simulink library "adv_mosfet"  (R2025b)
settings: Solver=VariableStepAuto  StartTime=0.0  StopTime=10.0  RelTol=1e-3
undefined symbols (not defined in the file): mosfet, Rgate_turn_off, Rgate_turn_on
libraries: fl_lib x8, nesl_utility x6, advanced_mosfet_lib x1
settings Model: Creator=dbagn  LastModifiedBy=dbagn

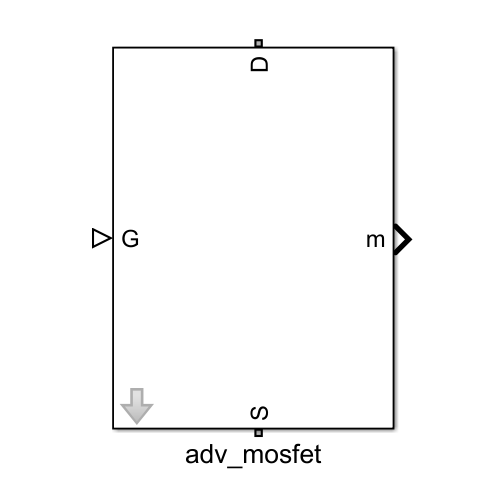
[thumbnail: Simulink's stored preview of the top-level diagram]
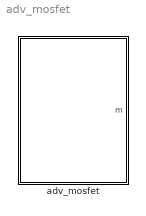
== system adv_mosfet ==
  adv_mosfet : Subsystem  mask{Rds_on_m=mosfet.inv.Rds_on, Vth_m=mosfet.inv.Vth, Vdon_diode_m=mosfet.inv.Vdon_diode, Rdon_diode_m=mosfet.inv.Rdon_diode, g_fs_m=mosfet.inv.g_fs, Cgs_m=mosfet.inv.Cgs, Cgd_m=mosfet.inv.Cgd, Cds_m=mosfet.inv.Cds, Eon_m=mosfet.inv.Eon, Eoff_m=mosfet.inv.Eoff, Err_m=mosfet.inv.Erec, Voff_sw_loss_m=mosfet.inv.Voff_sw_losses, Ion_sw_loss_m=mosfet.inv.Ion_sw_losses, Rgate_internal_m=mosfet.inv.Rgate_internal, Rgate_turn_on_m=Rgate_turn_on, Rgate_turn_off_m=Rgate_turn_off, Lstray_m=mosfet.inv.Lstray_module, Ld=mosfet.inv.Ld, RLd=mosfet.inv.RLd, Ls=mosfet.inv.Ls, RLs=mosfet.inv.RLs}
      mask prompts: Rds_on_m "Rds_on (Ohm)"; Vth_m "Vth (V)"; Vdon_diode_m "Vdon_diode (V)"; Rdon_diode_m "Rdon_diode (Ohm)"; g_fs_m "g_fs (A/V)"; Cgs_m "Cgs (F)"; Cgd_m "Cgd (F)"; Cds_m "Cds (F)"; Eon_m "Eon (J)"; Eoff_m "Eoff (J)"; Err_m "Err (J)"; Voff_sw_loss_m "Voff_sw_loss (V)"; Ion_sw_loss_m "Ion _sw_loss (A)"; Rgate_internal_m "Rgate internal (Ohm)"; Rgate_turn_on_m "Rgate turn on (Ohm)"; Rgate_turn_off_m "Rgate turn off (Ohm)"; Lstray_m "Lstray module (H)"; Ld "Ld (H)"; RLd "RLd (Ohm)"; Ls "Ls (H)"; RLs "RLs (Ohm)"
      settings: PortSchema="{\"entries\":[{\"content\":{\"sides\":[{\"content\":{\"connectorIds\":[\"LConn1\"]},\"type\":\"ConnectorPlacement.EquallySpacedRectSide\",\"uuid\":\"325dc963-858c-47f0-8995-f323ab4d9c46\"},{\"content\":{\"connectorIds\":[\"Out1\"],\"side\":\"RIGHT\"},\"type\":\"ConnectorPlacement.EquallySpacedRectSide\",\"uuid\":\"e9e66084-ecb2-40fb-9a1e-77677e0cc1df\"},{\"content\":{\"connectorIds\":[\"LConn2\"],\"side\":\"TOP\"},\"type\":\"ConnectorPlacement.EquallySpacedRectSide\",\"uuid\":\"9480d797-f2f6-459b-bb7c-d63861b57fde\"},{\"content\":{\"connectorIds\":[\"RConn1\"],\"side\":\"BOTTOM\"},\"type\":\"ConnectorPlacement.EquallySpacedRectSide\",\"uuid\":\"b13176d9-73b9-4822-9a0d-ec75065272bc\"}]},\"type\":\"ConnectorPlacement.EquallySpacedConnector\",\"uuid\":\"5e4a07d9-f5e8-4613-9049-5a866b5d2453\"}],\"packageUris\":[\"http://schema.mathworks.com/mf0/Connector/R2020b\"],\"version\":\"1.0\"}"

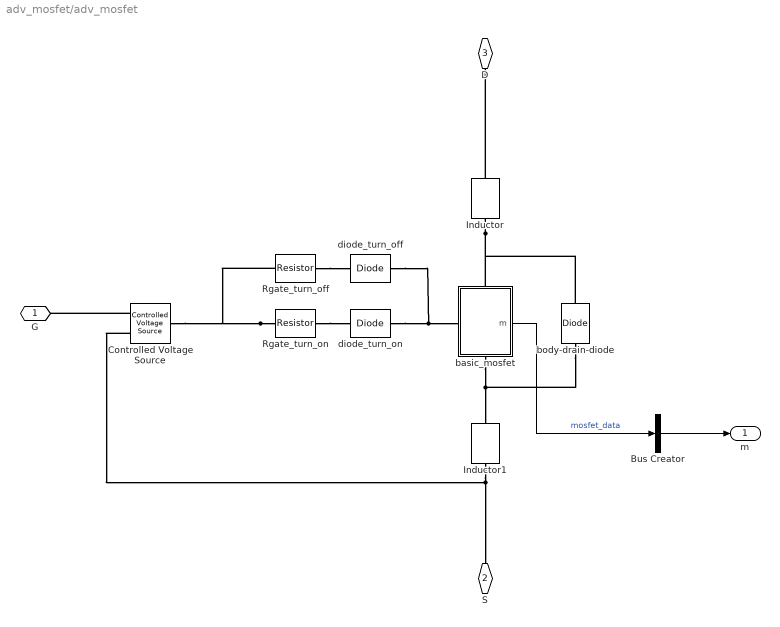
== system adv_mosfet/adv_mosfet ==
  Bus Creator : BusCreator  Inputs=1
  Controlled Voltage Source : fl_lib/Electrical/Electrical Sources/Controlled Voltage Source
  Inductor : fl_lib/Electrical/Electrical Elements/Inductor  l=Ld H  r=RLd Ohm  g=1e-9 1/Ohm  i_specify=off  i_priority=None  i=0 A  i_nominal_specify=off  i_nominal_value=1  i_nominal_unit=A  v_specify=off  v_priority=None  v=0 V  v_nominal_specify=off  v_nominal_value=1  v_nominal_unit=V  i_L_specify=off  i_L_priority=High  i_L=0 A  i_L_nominal_specify=off  i_L_nominal_value=1  i_L_nominal_unit=A
  Inductor1 : fl_lib/Electrical/Electrical Elements/Inductor  l=Ls H  r=RLs Ohm  g=1e-9 1/Ohm  i_specify=off  i_priority=None  i=0 A  i_nominal_specify=off  i_nominal_value=1  i_nominal_unit=A  v_specify=off  v_priority=None  v=0 V  v_nominal_specify=off  v_nominal_value=1  v_nominal_unit=V  i_L_specify=off  i_L_priority=High  i_L=0 A  i_L_nominal_specify=off  i_L_nominal_value=1  i_L_nominal_unit=A
  Rgate_turn_off : fl_lib/Electrical/Electrical Elements/Resistor  R=Rgate_turn_off_m Ohm  i_specify=off  i_priority=None  i=0 A  i_nominal_specify=off  i_nominal_value=1  i_nominal_unit=A  v_specify=off  v_priority=None  v=0 V  v_nominal_specify=off  v_nominal_value=1  v_nominal_unit=V
  Rgate_turn_on : fl_lib/Electrical/Electrical Elements/Resistor  R=Rgate_turn_on_m Ohm  i_specify=off  i_priority=None  i=0 A  i_nominal_specify=off  i_nominal_value=1  i_nominal_unit=A  v_specify=off  v_priority=None  v=0 V  v_nominal_specify=off  v_nominal_value=1  v_nominal_unit=V
  basic_mosfet : Subsystem  mask{Vth_m=Vth_m, Rds_on_m=Rds_on_m, g_fs_m=g_fs_m, Cgs_m=Cgs_m, Cgd_m=Cgd_m, Cds_m=Cds_m, Eon_m=Eon_m, Eoff_m=Eoff_m, Err_m=Err_m, Voff_sw_loss_m=Voff_sw_loss_m, Ion_sw_loss_m=Ion_sw_loss_m, Rgate_internal=Rgate_internal_m}
      mask prompts: Vth_m "Vth (V)"; Rds_on_m "Rds_on (Ohm)"; g_fs_m "g_fs (A/V)"; Cgs_m "Cgs (F)"; Cgd_m "Cgd (F)"; Cds_m "Cds (F)"; Eon_m "Eon (J)"; Eoff_m "Eoff (J)"; Err_m "Err (J)"; Voff_sw_loss_m "Voff_sw_loss (V)"; Ion_sw_loss_m "Ion_sw_loss (A)"; Rgate_internal "Rgate internal (Ohm)"
      settings: PortSchema="{\"entries\":[{\"content\":{\"sides\":[{\"content\":{\"connectorIds\":[\"LConn1\"]},\"type\":\"ConnectorPlacement.EquallySpacedRectSide\",\"uuid\":\"325dc963-858c-47f0-8995-f323ab4d9c46\"},{\"content\":{\"connectorIds\":[\"Out1\"],\"side\":\"RIGHT\"},\"type\":\"ConnectorPlacement.EquallySpacedRectSide\",\"uuid\":\"e9e66084-ecb2-40fb-9a1e-77677e0cc1df\"},{\"content\":{\"connectorIds\":[\"LConn2\"],\"side\":\"TOP\"},\"type\":\"ConnectorPlacement.EquallySpacedRectSide\",\"uuid\":\"9480d797-f2f6-459b-bb7c-d63861b57fde\"},{\"content\":{\"connectorIds\":[\"RConn1\"],\"side\":\"BOTTOM\"},\"type\":\"ConnectorPlacement.EquallySpacedRectSide\",\"uuid\":\"bd6f7c3f-e73f-43a3-8bfd-bc4aa1f2c71d\"}]},\"type\":\"ConnectorPlacement.EquallySpacedConnector\",\"uuid\":\"5e4a07d9-f5e8-4613-9049-5a866b5d2453\"}],\"packageUris\":[\"http://schema.mathworks.com/mf0/Connector/R2020b\"],\"version\":\"1.0\"}"
  body-drain-diode : fl_lib/Electrical/Electrical Elements/Diode  Vf=Vdon_diode_m V  Ron=Rdon_diode_m Ohm  Goff=1e-8 1/Ohm  i_specify=off  i_priority=None  i=0 A  i_nominal_specify=off  i_nominal_value=1  i_nominal_unit=A  v_specify=off  v_priority=None  v=0 V  v_nominal_specify=off  v_nominal_value=1  v_nominal_unit=V
  diode_turn_off : fl_lib/Electrical/Electrical Elements/Diode  Vf=0.35 V  Ron=Rdon_diode_m Ohm  Goff=1e-8 1/Ohm  i_specify=off  i_priority=None  i=0 A  i_nominal_specify=off  i_nominal_value=1  i_nominal_unit=A  v_specify=off  v_priority=None  v=0 V  v_nominal_specify=off  v_nominal_value=1  v_nominal_unit=V
  diode_turn_on : fl_lib/Electrical/Electrical Elements/Diode  Vf=0.35 V  Ron=Rdon_diode_m Ohm  Goff=1e-8 1/Ohm  i_specify=off  i_priority=None  i=0 A  i_nominal_specify=off  i_nominal_value=1  i_nominal_unit=A  v_specify=off  v_priority=None  v=0 V  v_nominal_specify=off  v_nominal_value=1  v_nominal_unit=V
  G : PMIOPort  Side=Left
  S : PMIOPort  Port=2  Side=Left
  D : PMIOPort  Port=3  Side=Right
  m : Outport
  wires:
  Bus Creator/1 -> m/1
  basic_mosfet/1(m) -> Bus Creator/1  "mosfet_data"
  connections:
  Rgate_turn_off/RConn1 -- diode_turn_off/RConn1
  Rgate_turn_on/RConn1 -- diode_turn_on/LConn1
  basic_mosfet/RConn1 -- Inductor1/LConn1 -- body-drain-diode/LConn1
  Controlled Voltage Source/RConn1 -- G/RConn1
  Rgate_turn_on/LConn1 -- Rgate_turn_off/LConn1 -- Controlled Voltage Source/LConn1
  diode_turn_on/RConn1 -- basic_mosfet/LConn1 -- diode_turn_off/LConn1
  Inductor/RConn1 -- basic_mosfet/LConn2 -- body-drain-diode/RConn1
  Controlled Voltage Source/RConn2 -- Inductor1/RConn1 -- S/RConn1
  Inductor/LConn1 -- D/RConn1

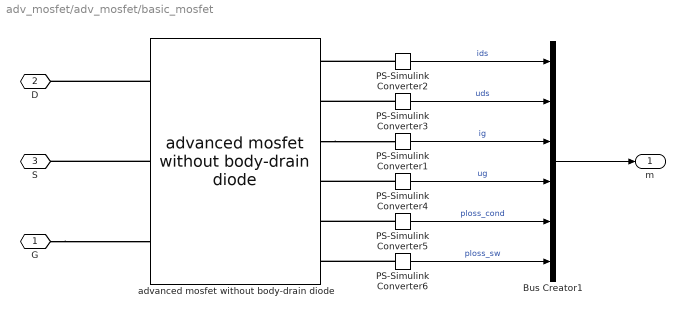
== system adv_mosfet/adv_mosfet/basic_mosfet ==
  Bus Creator1 : BusCreator  Inputs=6
  PS-Simulink Converter1 : nesl_utility/PS-Simulink Converter  PhysicalDomain=network_engine_domain  SubClassName=ps_output  LeftPortType=input  RightPortType=output  PseudoPeriodic=off  Frequencies=[]  VectorFormat=1-D array  Unit=A  AffineConversion=off
  PS-Simulink Converter2 : nesl_utility/PS-Simulink Converter  PhysicalDomain=network_engine_domain  SubClassName=ps_output  LeftPortType=input  RightPortType=output  PseudoPeriodic=off  Frequencies=[]  VectorFormat=1-D array  Unit=A  AffineConversion=off
  PS-Simulink Converter3 : nesl_utility/PS-Simulink Converter  PhysicalDomain=network_engine_domain  SubClassName=ps_output  LeftPortType=input  RightPortType=output  PseudoPeriodic=off  Frequencies=[]  VectorFormat=1-D array  Unit=V  AffineConversion=off
  PS-Simulink Converter4 : nesl_utility/PS-Simulink Converter  PhysicalDomain=network_engine_domain  SubClassName=ps_output  LeftPortType=input  RightPortType=output  PseudoPeriodic=off  Frequencies=[]  VectorFormat=1-D array  Unit=V  AffineConversion=off
  PS-Simulink Converter5 : nesl_utility/PS-Simulink Converter  PhysicalDomain=network_engine_domain  SubClassName=ps_output  LeftPortType=input  RightPortType=output  PseudoPeriodic=off  Frequencies=[]  VectorFormat=1-D array  Unit=W  AffineConversion=off
  PS-Simulink Converter6 : nesl_utility/PS-Simulink Converter  PhysicalDomain=network_engine_domain  SubClassName=ps_output  LeftPortType=input  RightPortType=output  PseudoPeriodic=off  Frequencies=[]  VectorFormat=1-D array  Unit=W  AffineConversion=off
  advanced mosfet without body-drain diode : advanced_mosfet_lib/advanced mosfet without body-drain diode  Vth=Vth_m V  g_fs=g_fs_m A/V  Rds_on=Rds_on_m Ohm  Cgs=Cgs_m F  Cgd=Cgd_m F  Cds=Cds_m F  Rg=Rgate_internal_m Ohm  Eon=Eon_m J  Eoff=Eoff_m J  Err=Err_m J  Voff_sw_loss=Voff_sw_loss_m V  Ion_sw_loss=Ion_sw_loss_m A  ids_i_specify=off  ids_i_priority=None  ids_i=0 A  ids_i_nominal_specify=off  ids_i_nominal_value=1  ids_i_nominal_unit=A  ids_ii_specify=off  ids_ii_priority=None  ids_ii=0 A  ids_ii_nominal_specify=off  ids_ii_nominal_value=1  ids_ii_nominal_unit=A  idsi_specify=off  idsi_priority=High  idsi=0 A  idsi_nominal_specify=off  idsi_nominal_value=1  idsi_nominal_unit=A  icgs_specify=off  icgs_priority=None  icgs=0 A  icgs_nominal_specify=off  icgs_nominal_value=1  icgs_nominal_unit=A  icgd_specify=off  icgd_priority=None  icgd=0 A  icgd_nominal_specify=off  icgd_nominal_value=1  icgd_nominal_unit=A  icds_specify=off  icds_priority=None  icds=0 A  icds_nominal_specify=off  icds_nominal_value=1  icds_nominal_unit=A  ugs_specify=off  ugs_priority=None  ugs=0 V  ugs_nominal_specify=off  ugs_nominal_value=1  ugs_nominal_unit=V  uds_specify=off  uds_priority=None  uds=0 V  uds_nominal_specify=off  uds_nominal_value=1  uds_nominal_unit=V  ucgs_specify=off  ucgs_priority=None  ucgs=0 V  ucgs_nominal_specify=off  ucgs_nominal_value=1  ucgs_nominal_unit=V  ucgd_specify=off  ucgd_priority=None  ucgd=0 V  ucgd_nominal_specify=off  ucgd_nominal_value=1  ucgd_nominal_unit=V  udsi_specify=off  udsi_priority=None  udsi=0 V  udsi_nominal_specify=off  udsi_nominal_value=1  udsi_nominal_unit=V  igs_specify=off  igs_priority=High  igs=0 A  igs_nominal_specify=off  igs_nominal_value=1  igs_nominal_unit=A  idsi_active_specify=off  idsi_active_priority=None  idsi_active=0 A  idsi_active_nominal_specify=off  idsi_active_nominal_value=1  idsi_active_nominal_unit=A  idsi_on_specify=off  idsi_on_priority=None  idsi_on=0 A  idsi_on_nominal_specify=off  idsi_on_nominal_value=1  idsi_on_nominal_unit=A
      settings: InternalSimscapePortConfiguration="{\"Bottom\":[],\"Left\":[{\"id\":\"D\",\"label\":\"D\",\"type\":\"foundation.electrical.electrical\"},{\"id\":\"S\",\"label\":\"S\",\"type\":\"foundation.electrical.electrical\"},{\"id\":\"G\",\"label\":\"G\",\"type\":\"foundation.electrical.electrical\"}],\"Right\":[{\"id\":\"idsi_out\",\"label\":\"ids\",\"type\":\"output\"},{\"id\":\"udsi_out\",\"label\":\"uds\",\"type\":\"output\"},{\"id\":\"igs_out\",\"label\":\"igs\",\"type\":\"output\"},{\"id\":\"ugs_out\",\"label\":\"ugs\",\"type\":\"output\"},{\"id\":\"ploss_cond\",\"label\":\"ploss_cond\",\"type\":\"output\"},{\"id\":\"ploss_sw\",\"label\":\"ploss_sw\",\"type\":\"output\"}],\"Top\":[]}"
  G : PMIOPort  Side=Left
  D : PMIOPort  Port=2  Side=Left
  S : PMIOPort  Port=3  Side=Right
  m : Outport
  wires:
  PS-Simulink Converter6/1 -> Bus Creator1/6  "ploss_sw"
  PS-Simulink Converter5/1 -> Bus Creator1/5  "ploss_cond"
  PS-Simulink Converter4/1 -> Bus Creator1/4  "ug"
  PS-Simulink Converter1/1 -> Bus Creator1/3  "ig"
  PS-Simulink Converter3/1 -> Bus Creator1/2  "uds"
  PS-Simulink Converter2/1 -> Bus Creator1/1  "ids"
  Bus Creator1/1 -> m/1
  connections:
  PS-Simulink Converter6/LConn1 -- advanced mosfet without body-drain diode/RConn6
  PS-Simulink Converter5/LConn1 -- advanced mosfet without body-drain diode/RConn5
  advanced mosfet without body-drain diode/RConn3 -- PS-Simulink Converter1/LConn1
  PS-Simulink Converter4/LConn1 -- advanced mosfet without body-drain diode/RConn4
  G/RConn1 -- advanced mosfet without body-drain diode/LConn3
  advanced mosfet without body-drain diode/LConn2 -- S/RConn1
  advanced mosfet without body-drain diode/LConn1 -- D/RConn1
  PS-Simulink Converter2/LConn1 -- advanced mosfet without body-drain diode/RConn1
  PS-Simulink Converter3/LConn1 -- advanced mosfet without body-drain diode/RConn2
